simulink model "SIM01_Discharge_cell"  (R2024a)
settings: Solver=ode1  StartTime=0.0  StopTime=2*3600  FixedStep=1e-2  MaxStep=1e-3  RelTol=1e-3
values from neighbouring files (symbols this model uses):
  A = 0.6*(PackFullChargeVoltage - PackExponentialZoneVoltage)    (= 1.44)    [COD01_BatteryCurve.m]
  B = (3/PackExponentialZoneCapacity)    (= 3)    [COD01_BatteryCurve.m]
  cellLPFTimeConstant = 30    [COD01_BatteryCurve.m]
  E0 = 0.9*(PackFullChargeVoltage + K - A + PackInternalResistance * PackNominalDischgCurrent)    [COD01_BatteryCurve.m]
  K = (3e-3)*(PackFullChargeVoltage - NominalPackVoltage + A*(exp(-B*NominalPackCapacity) - 1))*(PackRatedCapacity - NominalPackCapacity)/NominalPackCapacity    [COD01_BatteryCurve.m]
  n_parallel = 1    [COD01_BatteryCurve.m]
  n_series = 1    [COD01_BatteryCurve.m]
  PackRatedCapacity = cellRatedCapacity * n_parallel    (= 50)    [COD01_BatteryCurve.m]
  SOC_init = 1    [COD01_BatteryCurve.m]
settings Model: Creator=Dell PC  LastModifiedBy=Dell PC
settings SolverCC: AlgebraicLoopSolver=TrustRegion
settings DebuggingCC: UnconnectedInputMsg=warning  UnconnectedOutputMsg=warning  UnconnectedLineMsg=warning
settings ModelReferenceCC: EnableRefExpFcnMdlSchedulingChecks=on
settings RTWCC: GPUComputeCapability=3.5

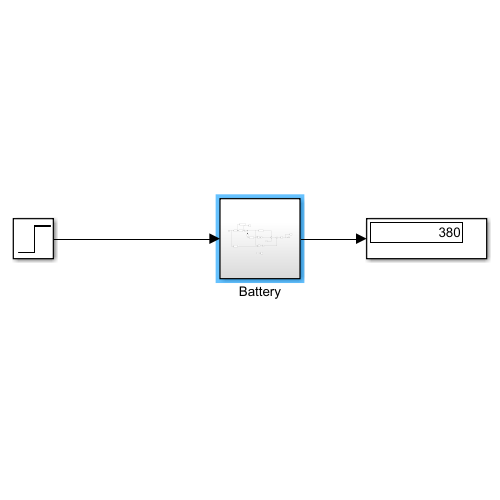
[thumbnail: Simulink's stored preview of the top-level diagram]
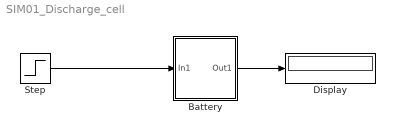
== system SIM01_Discharge_cell ==
  Battery : Subsystem
  Display : Display
  Step : Step  Time=0  After=25*n_parallel  SampleTime=0
  wires:
  Battery/1(Out1) -> Display/1
  Step/1 -> Battery/1(In1)

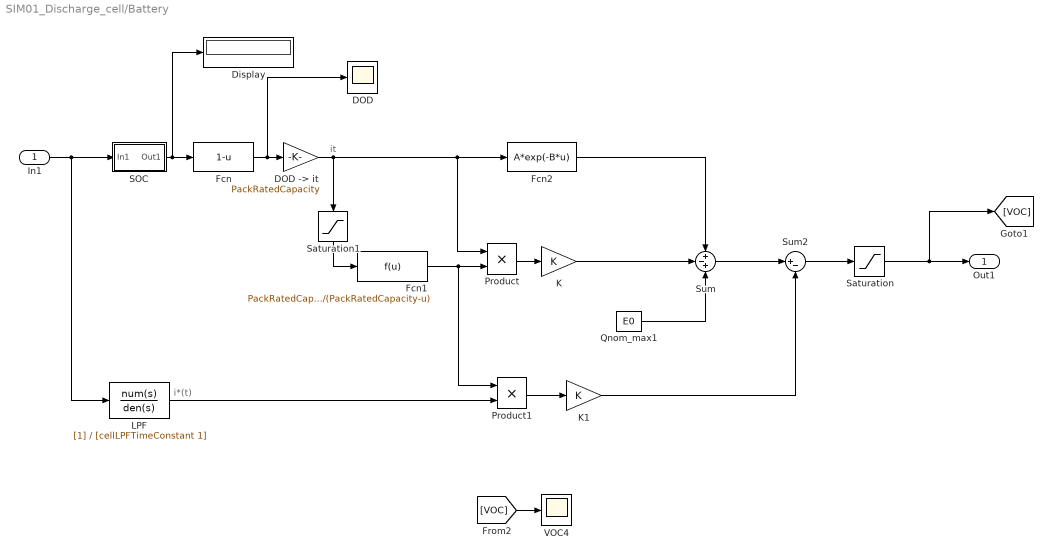
== system SIM01_Discharge_cell/Battery ==
  note: it
  note: i*(t)
  In1 : Inport
  DOD : Scope
  "DOD -> it" : Gain  Gain=PackRatedCapacity
  Display : Display
  Fcn : Fcn  Expr=1-u
  Fcn1 : Fcn  Expr=PackRatedCapacity/(PackRatedCapacity-u)
  Fcn2 : Fcn  Expr=A*exp(-B*u)
  K : Gain  Gain=K
  K1 : Gain  Gain=K
  LPF : TransferFcn  Denominator=[cellLPFTimeConstant 1]
  Product : Product
  Product1 : Product
  Qnom_max1 : Constant  Value=E0
  SOC : Subsystem
  Saturation : Saturate  UpperLimit=inf  LowerLimit=30*n_series
  Saturation1 : Saturate  UpperLimit=PackRatedCapacity*(1-1e-6)  LowerLimit=0
  Sum : Sum  Inputs=+-+
  Sum2 : Sum  Inputs=|+-
  VOC4 : Scope
  Out1 : Outport
  wires:
  K/1 -> Sum/2
  Fcn1/1 -> Product/2, Product1/1
  Product/1 -> K/1
  Saturation/1 -> [VOC], Out1/1
  Sum2/1 -> Saturation/1
  "DOD -> it"/1 -> Saturation1/1, Fcn2/1, Product/1
  Qnom_max1/1 -> Sum/3
  SOC/1(Out1) -> Fcn/1, Display/1
  Sum/1 -> Sum2/1
  Fcn2/1 -> Sum/1
  Product1/1 -> K1/1
  LPF/1 -> Product1/2
  In1/1 -> LPF/1, SOC/1(In1)
  K1/1 -> Sum2/2
  Fcn/1 -> DOD/1, "DOD -> it"/1
  Saturation1/1 -> Fcn1/1
  [VOC] -> VOC4/1

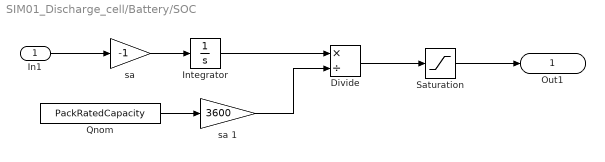
== system SIM01_Discharge_cell/Battery/SOC ==
  In1 : Inport
  Divide : Product  Inputs=*/
  Integrator : Integrator  InitialCondition=PackRatedCapacity*SOC_init*3600  LimitOutput=on  UpperSaturationLimit=PackRatedCapacity*3600  LowerSaturationLimit=0
  Qnom : Constant  Value=PackRatedCapacity
  Saturation : Saturate  UpperLimit=1-1e-6  LowerLimit=0+1e-6
  "sa " : Gain  Gain=-1
  sa 1 : Gain  Gain=3600
  Out1 : Outport
  wires:
  Qnom/1 -> sa 1/1
  Saturation/1 -> Out1/1
  In1/1 -> "sa "/1
  "sa "/1 -> Integrator/1
  Integrator/1 -> Divide/1
  sa 1/1 -> Divide/2
  Divide/1 -> Saturation/1
